simulink model "crane"  (R2015a)
settings: Solver=ode45  StartTime=0.0  StopTime=100.0  RelTol=1e-3
undefined symbols (not defined in the file or in its folder): Gr, rr
libraries: cstblocks x3
settings Model: Creator=roevhat  LastModifiedBy=lbromo12

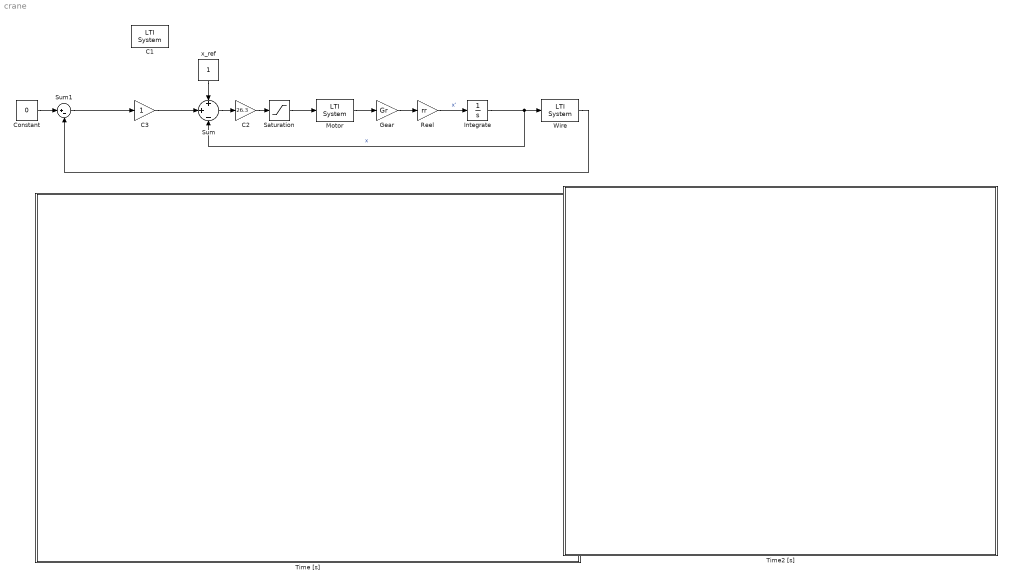
== system crane ==
  C1 : cstblocks/LTI System  sys=C1  IC=[]
  C2 : Gain  Gain=26.3
  C3 : Gain
  Constant : Constant  Value=0
  Gear : Gain  Gain=Gr
  Integrate : Integrator
  Motor : cstblocks/LTI System  sys=M  IC=[]
  "Reel " : Gain  Gain=rr
  Saturation : Saturate  UpperLimit=14  LowerLimit=-14
  Sum : Sum  Inputs=+|+|-
  Sum1 : Sum  Inputs=|+-
  Time [s] : Subsystem  DialogController=hmiCreateDDGDialog  IsWebBlock=on  mask(MathWorksWebBlock){webBlockId=2ac42065-2a1d-45d8-b9d1-76f78bc34ac1, webBlockType=sdiscope, ShowInitialText=on, HMISrcModelName=[]}
      mask prompts: webBlockId "WebBlock Id"; webBlockType "WebBlock Type"; HMISrcModelName "Source Model"
      mask Help: helpview([docroot '/mapfiles/simulink.map'], 'hmi_scope')
      mask Display:
      | if strcmp(get_param(bdroot(gcb),'BlockDiagramType'), 'library')
      |     image([(matlabroot) '/toolbox/simulink/hmi/icons/DashboardScope.png']);
      | end
  Time2 [s] : Subsystem  DialogController=hmiCreateDDGDialog  IsWebBlock=on  mask(MathWorksWebBlock){webBlockId=92e58269-1bcc-4d94-8be3-c2f5956555b2, webBlockType=sdiscope, ShowInitialText=on, HMISrcModelName=[]}
      mask prompts: webBlockId "WebBlock Id"; webBlockType "WebBlock Type"; HMISrcModelName "Source Model"
      mask Help: helpview([docroot '/mapfiles/simulink.map'], 'hmi_scope')
      mask Display:
      | if strcmp(get_param(bdroot(gcb),'BlockDiagramType'), 'library')
      |     image([(matlabroot) '/toolbox/simulink/hmi/icons/DashboardScope.png']);
      | end
  Wire : cstblocks/LTI System  sys=W  IC=[]
  x_ref : Constant
  wires:
  Integrate/1 -> Sum/3, Wire/1  "x"
  Motor/1 -> Gear/1
  Gear/1 -> "Reel "/1
  "Reel "/1 -> Integrate/1  "x'"
  Wire/1 -> Sum1/2
  Sum/1 -> C2/1
  Constant/1 -> Sum1/1
  x_ref/1 -> Sum/1
  Sum1/1 -> C3/1
  C2/1 -> Saturation/1
  Saturation/1 -> Motor/1
  C3/1 -> Sum/2

== system crane/Time [s] ==

== system crane/Time2 [s] ==
